simulink model "coffee"  (R2017a)
settings: Solver=FixedStepDiscrete  StartTime=0.0  StopTime=30  FixedStep=0.1  RelTol=1e-3  EnableMultiTasking=on
settings Model: Creator=thr  LastModifiedBy=thr
settings SolverCC: AutoInsertRateTranBlk=on
settings DataIOCC: LimitDataPoints=on
settings OptimizationCC: LifeSpan=inf
settings DebuggingCC: AllowSymbolicDim=off  SFUnexpectedBacktrackingDiag=warning  SFNoUnconditionalDefaultTransitionDiag=warning  SFExecutionAtInitializationDiag=none
settings GRTTargetCC: TargetLangStandard=C89/C90 (ANSI)  GeneratePreprocessorConditionals=Disable all
settings ConfigComp: CovMetricSettings=dw  CovHtmlReporting=on  CovSaveCumulativeToWorkspaceVar=on  CovSaveSingleToWorkspaceVar=on  CovShowResultsExplorer=off  CovExternalEMLEnable=off  CovSFcnEnable=off

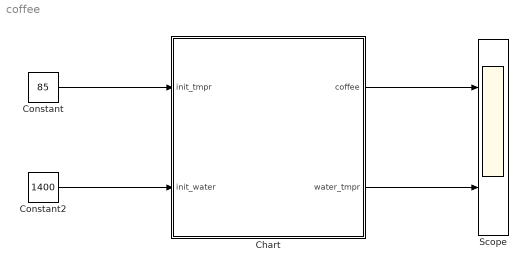
== system coffee ==
  Chart : Stateflow chart  TreatAsAtomicUnit=on
  Constant : Constant  Value=85  OutDataTypeStr=int32
  Constant2 : Constant  Value=1400  OutDataTypeStr=int32
  Scope : Scope  NumInputPorts=2
  wires:
  Constant/1 -> Chart/1(init_tmpr)
  Constant2/1 -> Chart/2(init_water)
  Chart/1(coffee) -> Scope/1
  Chart/2(water_tmpr) -> Scope/2

== stateflow chart coffee/Chart ==
  state OFF
    entry:
    coffee = 0;
    water = init_water
    fprintf('OFF')
  state ON
    entry:
    water_tmpr = init_tmpr;
    state HEATING
      entry: water_tmpr = water_tmpr + 10;
    state FILLING_CARAFE
      exit: water=water-20;
      coffee=coffee+20;
    state BEEPING
    (default) -> HEATING : {fprintf('HEATING')}
    HEATING -> HEATING [order 2] : after(1, sec)
        | {fprintf('HEATING'),
        |  fprintf('<- water_tmpr - %d', water_tmpr)}
    HEATING -> FILLING_CARAFE [order 1] : [water_tmpr >=100]
        | {fprintf('FILLING_CARAFE')}
    FILLING_CARAFE -> FILLING_CARAFE [order 2] : after(1, sec)
        | {fprintf('FILLING_CARAFE'),
        |  fprintf('<- coffee - %d', coffee)}
    FILLING_CARAFE -> BEEPING [order 1] : [coffee>=100]
        | {fprintf('BEEPING'),
        | fprintf('<- coffee - %d', coffee),
        | fprintf('<- water - %d', water)}
  state STANDBY
  (default) -> OFF
  OFF -> ON : [water >= 100]
  ON -> OFF : [water < 100]
  BEEPING -> STANDBY : after(3, sec)
      | {fprintf('STANDBY')}
  data: coffee output int32; water_tmpr output int32; init_tmpr input int32; water local int32; init_water input int32
